simulink model "processo_fig_7_7_b_NISE_rampa"  (R2017b)
settings: Solver=VariableStepAuto  StartTime=0.0  StopTime=5  RelTol=1e-3
libraries: simulink x1
settings Model: Creator=fernandopassold  LastModifiedBy=fernandopassold
settings CodeAppCC: StateflowObjectComments=on

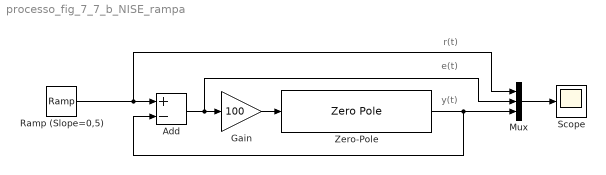
== system processo_fig_7_7_b_NISE_rampa ==
  note: y(t)
  note: e(t)
  note: r(t)
  Add : Sum  Inputs=+-
  Gain : Gain  Gain=100
  Mux : Mux  Inputs=3
  Ramp (Slope=0,5) : simulink/Sources/Ramp  slope=0.5  start=1  X0=0
  Scope : Scope
  Zero-Pole : ZeroPole  Zeros=[-2 -5 -6]  Poles=[0 -8 -10 -12]
  wires:
  Mux/1 -> Scope/1
  Add/1 -> Mux/2, Gain/1
  Ramp (Slope=0,5)/1 -> Mux/1, Add/1
  Gain/1 -> Zero-Pole/1
  Zero-Pole/1 -> Add/2, Mux/3
